simulink model "BasicTestModel"  (R2015a)
settings: Solver=ode3  StartTime=0.0  StopTime=10.0  FixedStep=1/200  RelTol=1e-3
undefined symbols (not defined in the file): i
libraries: PoliArd x8
settings Model: ExtModeTrigDuration=2  Creator=User  LastModifiedBy=user
settings OptimizationCC: OptimizeModelRefInitCode=on  LifeSpan=1
settings DebuggingCC: UnderspecifiedInitializationDetection=Classic  MergeDetectMultiDrivingBlocksExec=none
settings HardwareCC: ProdLargestAtomicInteger=Long  ProdLargestAtomicFloat=Double  ProdEndianess=LittleEndian  ProdHWDeviceType=ARM Compatible->ARM Cortex
settings RTWCC: SystemTargetFile=realtime.tlc  GenerateMakefile=off  TemplateMakefile=realtime.tmf  Description=Run on Target Hardware  RTWVerbose=off
settings ERTTargetCC: CombineOutputUpdateFcns=off  ExtModeTransport=3  ExtModeMexFile=ext_serial_win32_comm_rtt  ExtModeMexArgs=0 1 9600  ERTSrcFileBannerTemplate=realtime_code_template.cgt  ERTHdrFileBannerTemplate=realtime_code_template.cgt  ERTDataSrcFileTemplate=realtime_code_template.cgt  ERTDataHdrFileTemplate=realtime_code_template.cgt  ERTCustomFileTemplate=realtime_file_process.tlc

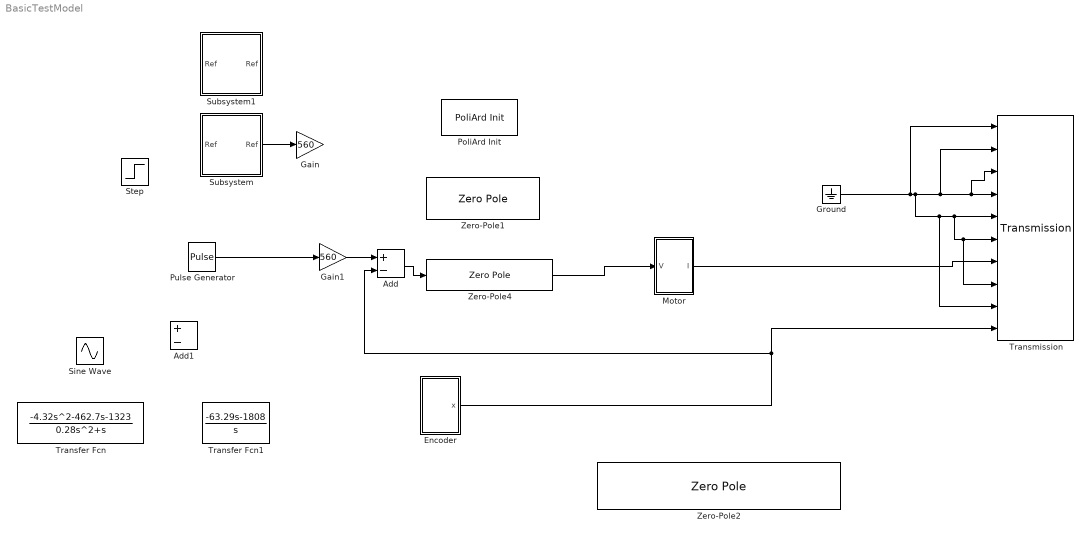
== system BasicTestModel ==
  Add : Sum  Inputs=+-
  Add1 : Sum  Inputs=+-
  "Encoder " : Subsystem
  Gain : Gain  Gain=560
  Gain1 : Gain  Gain=560
  Ground : Ground
  Motor : Subsystem
  PoliArd Init : PoliArd/PoliArd Init
  Pulse Generator : DiscretePulseGenerator  PulseType=Time based  Amplitude=2  Period=10  PulseWidth=50  PhaseDelay=5
  Sine Wave : Sin  Amplitude=2  SampleTime=0
  Step : Step  SampleTime=0
  Subsystem : Subsystem
  Subsystem1 : Subsystem
  Transfer Fcn : TransferFcn  Numerator=[-4.32 -462.7 -1323]  Denominator=[0.28 1 0]
  Transfer Fcn1 : TransferFcn  Numerator=[-63.29 -1808]  Denominator=[1 0]
  Transmission : PoliArd/Transmission  sample_freq=200  sig_to_send=6
  Zero-Pole1 : ZeroPole  Zeros=[-5+22i, -5-22i]  Poles=[0, -100]  Gain=-0.03
  Zero-Pole2 : ZeroPole  Zeros=[-79.8,-33.1, -58.4+16.9*i , -58.4-16.9*i]  Poles=[0,-111,-566+45.7*i, -566-45.7*i]  Gain=-4.3815
  Zero-Pole4 : ZeroPole  Zeros=[9.52+3.16i,9.52-3.16i]  Poles=[0,-100]  Gain=-0.016498
  wires:
  Ground/1 -> Transmission/1, Transmission/9, Transmission/8, Transmission/6, Transmission/5, Transmission/2, Transmission/3, Transmission/4
  "Encoder "/1(x) -> Transmission/10, Add/2
  Subsystem/1("Ref ") -> Gain/1
  Gain1/1 -> Add/1
  Motor/1(I) -> Transmission/7
  Add/1 -> Zero-Pole4/1
  Pulse Generator/1 -> Gain1/1
  Zero-Pole4/1 -> Motor/1(V)

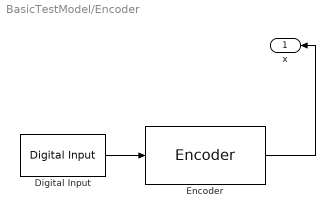
== system BasicTestModel/Encoder  ==
  Digital Input : PoliArd/Digital Input  DI_pin=2  DIsample=1/200
  Encoder : PoliArd/Encoder  EncoderID=1  dt_enc=-1
  x : Outport
  wires:
  Digital Input/1 -> Encoder/1
  Encoder/1 -> x/1

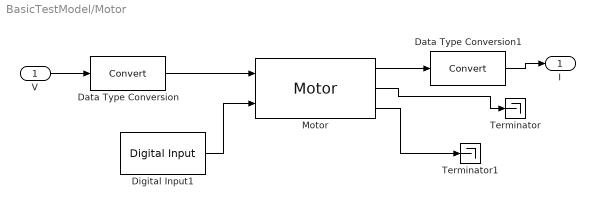
== system BasicTestModel/Motor ==
  V : Inport
  Data Type Conversion : DataTypeConversion
  Data Type Conversion1 : DataTypeConversion
  Digital Input1 : PoliArd/Digital Input  DI_pin=3  DIsample=1/200
  Motor : PoliArd/Motor  MotorID=1  DC_bus_mask=12  dt_mot=1/200
  Terminator : Terminator
  Terminator1 : Terminator
  I : Outport
  wires:
  Data Type Conversion/1 -> Motor/1
  Digital Input1/1 -> Motor/2
  V/1 -> Data Type Conversion/1
  Motor/3 -> Terminator1/1
  Motor/2 -> Terminator/1
  Motor/1 -> Data Type Conversion1/1
  Data Type Conversion1/1 -> I/1

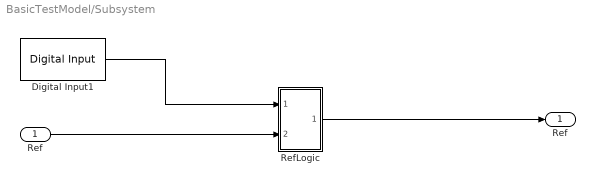
== system BasicTestModel/Subsystem ==
  Ref : Inport
  Digital Input1 : PoliArd/Digital Input  DI_pin=3  DIsample=1/200
  RefLogic : Subsystem
  "Ref " : Outport
  wires:
  Digital Input1/1 -> RefLogic/1(In1)
  Ref/1 -> RefLogic/2(In2)
  RefLogic/1(Out1) -> "Ref "/1

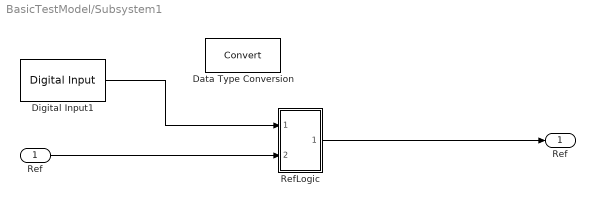
== system BasicTestModel/Subsystem1 ==
  Ref : Inport
  Data Type Conversion : DataTypeConversion
  Digital Input1 : PoliArd/Digital Input  DI_pin=3  DIsample=1/200
  RefLogic : Subsystem
  "Ref " : Outport
  wires:
  Digital Input1/1 -> RefLogic/1(In1)
  Ref/1 -> RefLogic/2(In2)
  RefLogic/1(Out1) -> "Ref "/1

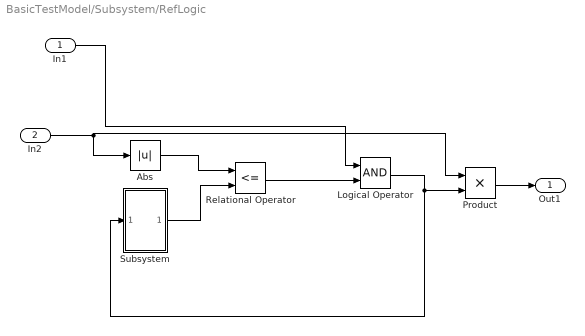
== system BasicTestModel/Subsystem/RefLogic ==
  In1 : Inport
  In2 : Inport  Port=2
  Abs : Abs
  Logical Operator : Logic  AllPortsSameDT=off  OutDataTypeStr=boolean
  Product : Product
  Relational Operator : RelationalOperator  Operator=<=  OutDataTypeStr=boolean
  Subsystem : Subsystem
  Out1 : Outport
  wires:
  In2/1 -> Abs/1, Product/1
  Product/1 -> Out1/1
  Logical Operator/1 -> Product/2, Subsystem/1(In1)
  Subsystem/1(Out1) -> Relational Operator/2
  Relational Operator/1 -> Logical Operator/2
  In1/1 -> Logical Operator/1
  Abs/1 -> Relational Operator/1

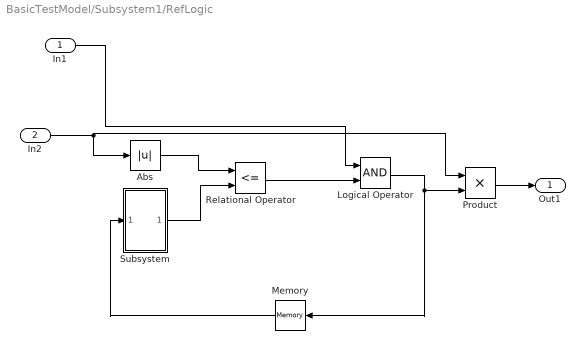
== system BasicTestModel/Subsystem1/RefLogic ==
  In1 : Inport
  In2 : Inport  Port=2
  Abs : Abs
  Logical Operator : Logic  AllPortsSameDT=off  OutDataTypeStr=boolean
  Memory : Memory
  Product : Product
  Relational Operator : RelationalOperator  Operator=<=  OutDataTypeStr=boolean
  Subsystem : Subsystem
  Out1 : Outport
  wires:
  In2/1 -> Abs/1, Product/1
  Product/1 -> Out1/1
  Logical Operator/1 -> Product/2, Memory/1
  Subsystem/1(Out1) -> Relational Operator/2
  Relational Operator/1 -> Logical Operator/2
  In1/1 -> Logical Operator/1
  Abs/1 -> Relational Operator/1
  Memory/1 -> Subsystem/1(In1)

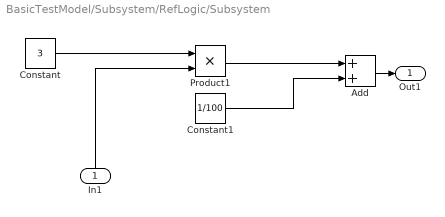
== system BasicTestModel/Subsystem/RefLogic/Subsystem ==
  In1 : Inport
  Add : Sum
  Constant : Constant  Value=3
  Constant1 : Constant  Value=1/100
  Product1 : Product
  Out1 : Outport
  wires:
  Product1/1 -> Add/1
  In1/1 -> Product1/2
  Add/1 -> Out1/1
  Constant1/1 -> Add/2
  Constant/1 -> Product1/1

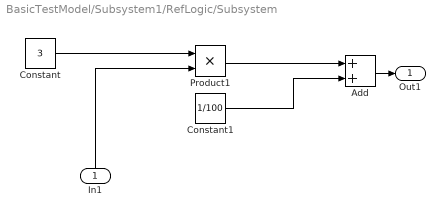
== system BasicTestModel/Subsystem1/RefLogic/Subsystem ==
  In1 : Inport
  Add : Sum
  Constant : Constant  Value=3
  Constant1 : Constant  Value=1/100
  Product1 : Product
  Out1 : Outport
  wires:
  Product1/1 -> Add/1
  In1/1 -> Product1/2
  Add/1 -> Out1/1
  Constant1/1 -> Add/2
  Constant/1 -> Product1/1
